simulink model "MLIB_ShBiSat_BAM_F32"  (Simulink 7.3)
settings: Solver=ode45  StartTime=0.0  StopTime=10.0  RelTol=1e-3
settings Model: Creator=B17364  LastModifiedBy=B17364

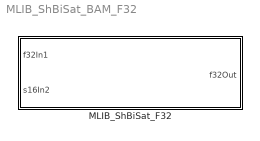
== system MLIB_ShBiSat_BAM_F32 ==
  MLIB_ShBiSat_F32 : Subsystem  mask(MLIB_ShBiSat_F32){}
      mask help: Bit accurate model of the fuction shifts the first parameter to left or right by number defined by second parameter and saturate if necessary. If the sign of second parameter is negative, shift to right. All parameters as well as input and output are 32bit integers.
      mask init:
      | pos = get_param(gcb, 'Position');width = pos(3) - pos(1); height = pos(4) - pos(2);tX=width/2;tY=height*0.9;
      mask Display: color('black');port_label('input',1,'f32In1');port_label('input',2,'s16In2');port_label('output',1,'f32Out');color('black');disp('MLIB_ShBiSat_F32');color('blue');text(tX,tY, 'BAM', 'horizontalAlignment', 'center');

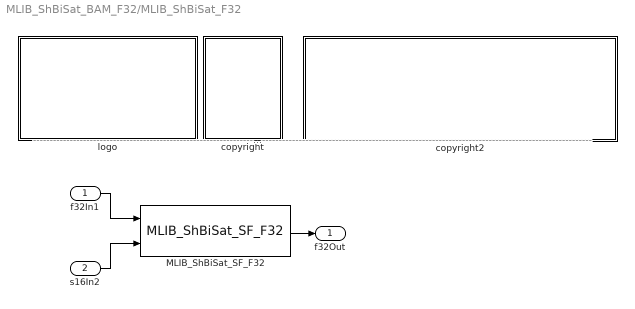
== system MLIB_ShBiSat_BAM_F32/MLIB_ShBiSat_F32 ==
  note: ---------------------------------------------------------------------------------------------------------------------------------------------------------------------------------------------------
  f32In1 : Inport  OutDataType=fixdt(1, 16)  OutScaling=2^0
  s16In2 : Inport  Port=2  OutDataType=fixdt(1, 16)  OutScaling=2^0
  MLIB_ShBiSat_SF_F32 : S-Function  FunctionName=MLIB_ShBiSat_SF_F32  EnableBusSupport=off
  copyright : Subsystem
      mask Display: text(10,90,'FILE:');text(10,75,'DESRIPTION:')text(10,60,'COPYRIGHT:')text(10,45,'VERSION:')text(10,30,'DATE:')
  copyright2 : Subsystem
      mask Display: text(10,90,'MLIB_ShBiSat_BAM_F32.mdl');text(10,75,'Shift the first parameter to left or right and saturate if necessary.');text(10,60,'Freescale')text(10,45,'0.1');text(10,30,'26-Aug-2011');
  logo : Subsystem
      mask Display: image(imread('logo.jpg'))
  f32Out : Outport  OutDataType=fixdt(1, 16)  OutScaling=2^0
  wires:
  f32In1/1 -> MLIB_ShBiSat_SF_F32/1
  s16In2/1 -> MLIB_ShBiSat_SF_F32/2
  MLIB_ShBiSat_SF_F32/1 -> f32Out/1

== system MLIB_ShBiSat_BAM_F32/MLIB_ShBiSat_F32/copyright ==

== system MLIB_ShBiSat_BAM_F32/MLIB_ShBiSat_F32/copyright2 ==

== system MLIB_ShBiSat_BAM_F32/MLIB_ShBiSat_F32/logo ==
